simulink library "avionics_T2_lib"  (Simulink 6.6)
undefined symbols (not defined in the file or in its folder): EngineID, Timestep
libraries: aeroutilslib x3, Telemetry_Lib x3, Calibration_Lib x2, simulink x1
settings Model: Creator=amurch  LastModifiedBy=amurch

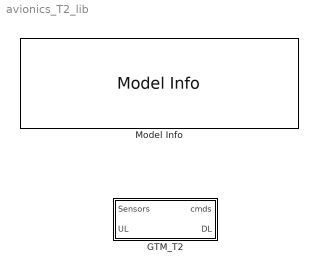
== system avionics_T2_lib ==
  GTM_T2 : Subsystem
  Model Info : simulink/Model-Wide Utilities/Model Info  SystemSampleTime=-1  InitialBlockCM=None  BlockCM=None  Frame=on  DisplayStringWithTags=|  HorizontalTextAlignment=Center  LeftAlignmentValue=0.5  SourceBlockDiagram=avionics_T2_lib  TagMaxNumber=20
      | GTM T2 Avionics Library
      | %<ModelVersion>
      | Las modified by %<LastModifiedBy> on %<LastModificationDate>

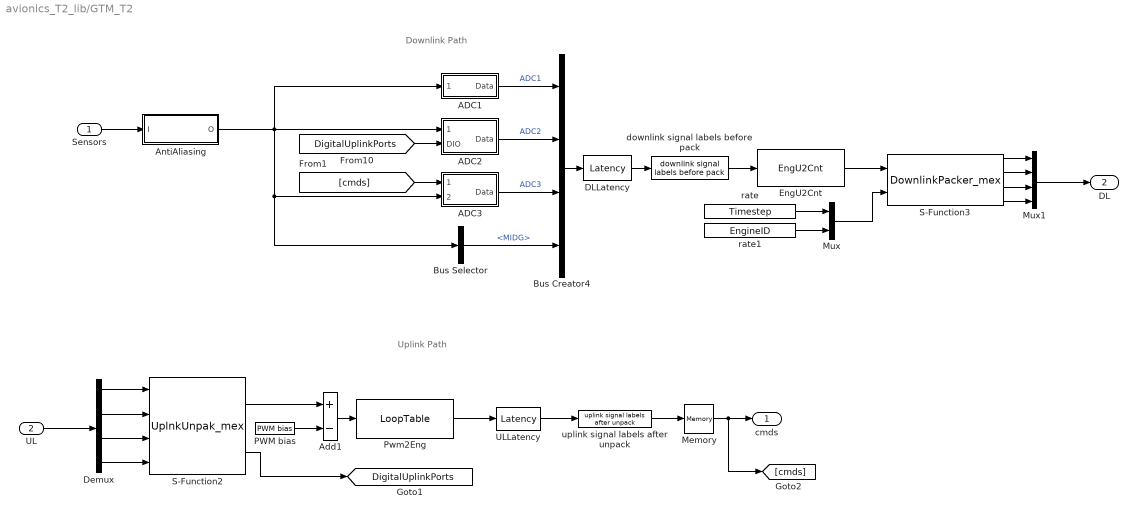
== system avionics_T2_lib/GTM_T2 ==
  note: Downlink Path
  note: Uplink Path
  Sensors : Inport
  UL : Inport  Port=2
  ADC1 : Subsystem
  ADC2 : Subsystem
  ADC3 : Subsystem
  Add1 : Sum  Inputs=+-  OutScaling=2^-10
  AntiAliasing : Subsystem
  Bus Creator4 : BusCreator
  Bus Selector : BusSelector  OutputSignals=MIDG
  DLLatency : aeroutilslib/Latency  SystemSampleTime=-1  Latency=.01  timestep=Timestep
  Demux : Demux
  EngU2Cnt : Calibration_Lib/EngU2Cnt  SystemSampleTime=-1
  Memory : Memory
  Mux : Mux  Inputs=2
  Mux1 : Mux
  PWM bias : Telemetry_Lib/PWM bias  SystemSampleTime=-1
  Pwm2Eng : Calibration_Lib/LoopTable  SystemSampleTime=-1  XTable=UpCals_Pwm  YTable=UpCals_Eng
  S-Function2 : S-Function  FunctionName=UplnkUnpak_mex
  S-Function3 : S-Function  FunctionName=DownlinkPacker_mex
  ULLatency : aeroutilslib/Latency  SystemSampleTime=-1  Latency=.01  timestep=Timestep
  downlink signal labels before pack : Telemetry_Lib/downlink signal labels before pack  SystemSampleTime=-1
  rate : Constant  Value=Timestep
  rate1 : Constant  Value=EngineID
  uplink signal labels after unpack : Telemetry_Lib/uplink signal labels after unpack  SystemSampleTime=-1
  cmds : Outport
  DL : Outport  Port=2
  tag scope: DigitalUplinkPorts=global
  wires:
  S-Function2/1 -> Add1/1
  Add1/1 -> Pwm2Eng/1
  PWM bias/1 -> Add1/2
  [cmds] -> ADC3/1(cmds)
  [DigitalUplinkPorts] -> ADC2/2(DIO)
  DLLatency/1 -> downlink signal labels before pack/1
  downlink signal labels before pack/1 -> EngU2Cnt/1
  ULLatency/1 -> uplink signal labels after unpack/1
  Memory/1 -> [cmds], cmds/1
  Bus Creator4/1 -> DLLatency/1
  Bus Selector/1 -> Bus Creator4/4  "<MIDG>"
  AntiAliasing/1(O) -> Bus Selector/1, ADC3/2(ADC3), ADC2/1(ADC2), ADC1/1(ADC1)
  ADC3/1(Data) -> Bus Creator4/3  "ADC3"
  ADC2/1(Data) -> Bus Creator4/2  "ADC2"
  ADC1/1(Data) -> Bus Creator4/1  "ADC1"
  UL/1 -> Demux/1
  Demux/4 -> S-Function2/4
  Demux/3 -> S-Function2/3
  Demux/2 -> S-Function2/2
  Demux/1 -> S-Function2/1
  uplink signal labels after unpack/1 -> Memory/1
  Pwm2Eng/1 -> ULLatency/1
  S-Function2/2 -> [DigitalUplinkPorts]
  Mux1/1 -> DL/1
  S-Function3/4 -> Mux1/4
  S-Function3/3 -> Mux1/3
  S-Function3/2 -> Mux1/2
  S-Function3/1 -> Mux1/1
  Mux/1 -> S-Function3/2
  rate1/1 -> Mux/2
  rate/1 -> Mux/1
  EngU2Cnt/1 -> S-Function3/1
  Sensors/1 -> AntiAliasing/1(I)

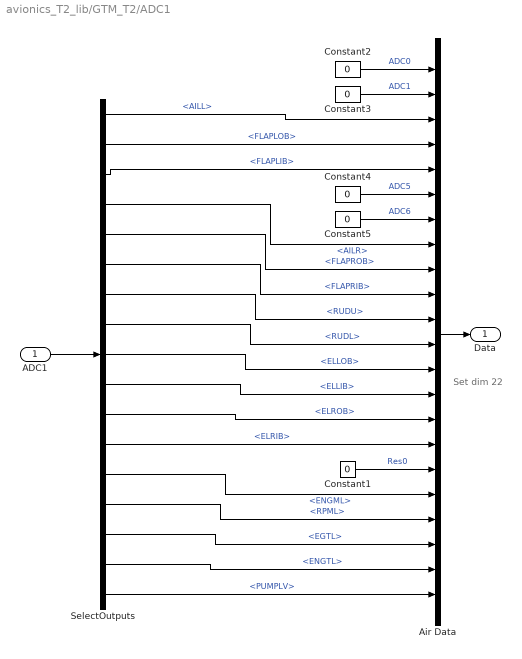
== system avionics_T2_lib/GTM_T2/ADC1 ==
  note: Set dim 22
  ADC1 : Inport
  Air Data : BusCreator  Inputs=22
  Constant{1..5} (5 alike) : Constant  Value=0
  SelectOutputs : BusSelector  OutputSignals=Pots.AILL,Pots.FLAPLOB,Pots.FLAPLIB,Pots.AILR,Pots.FLAPROB,Pots.FLAPRIB,Pots.RUDU,Pots.RUDL,Pots.ELLOB,Pots.ELLIB,Pots.ELROB,Pots.ELRIB,ECUL.ENGML,ECUL.RPML,ECUL.EGTL,ECUL.ENGTL,ECUL.PUMPLV
  Data : Outport  PortDimensions=22
  wires:
  SelectOutputs/17 -> Air Data/22  "<PUMPLV>"
  SelectOutputs/16 -> Air Data/21  "<ENGTL>"
  SelectOutputs/15 -> Air Data/20  "<EGTL>"
  SelectOutputs/14 -> Air Data/19  "<RPML>"
  SelectOutputs/13 -> Air Data/18  "<ENGML>"
  SelectOutputs/12 -> Air Data/16  "<ELRIB>"
  SelectOutputs/11 -> Air Data/15  "<ELROB>"
  SelectOutputs/10 -> Air Data/14  "<ELLIB>"
  SelectOutputs/9 -> Air Data/13  "<ELLOB>"
  SelectOutputs/8 -> Air Data/12  "<RUDL>"
  SelectOutputs/7 -> Air Data/11  "<RUDU>"
  SelectOutputs/6 -> Air Data/10  "<FLAPRIB>"
  SelectOutputs/5 -> Air Data/9  "<FLAPROB>"
  SelectOutputs/4 -> Air Data/8  "<AILR>"
  SelectOutputs/3 -> Air Data/5  "<FLAPLIB>"
  SelectOutputs/2 -> Air Data/4  "<FLAPLOB>"
  SelectOutputs/1 -> Air Data/3  "<AILL>"
  Constant5/1 -> Air Data/7  "ADC6"
  Constant4/1 -> Air Data/6  "ADC5"
  Constant3/1 -> Air Data/2  "ADC1"
  Constant2/1 -> Air Data/1  "ADC0"
  ADC1/1 -> SelectOutputs/1
  Air Data/1 -> Data/1
  Constant1/1 -> Air Data/17  "Res0"

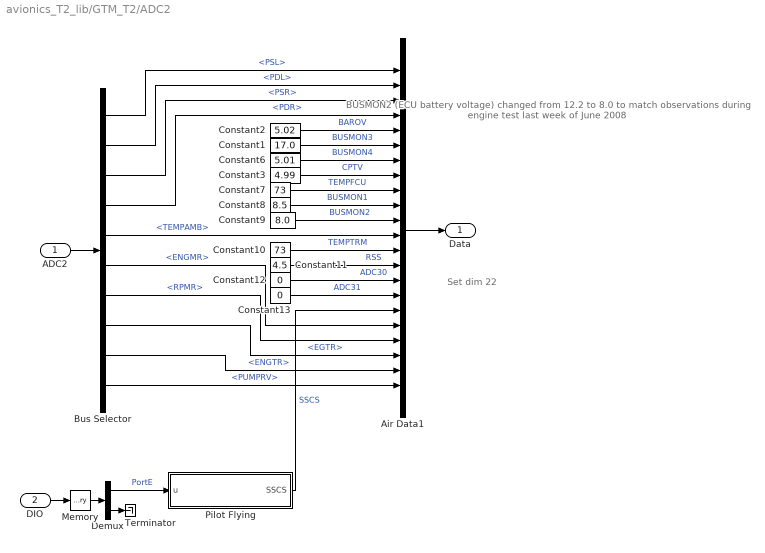
== system avionics_T2_lib/GTM_T2/ADC2 ==
  note: Set dim 22
  note: BUSMON2 (ECU battery voltage)
      | changed from 12.2 to 8.0 to
      | match observations during engine test
      | last week of June 2008
  ADC2 : Inport
  DIO : Inport  Port=2
  Air Data1 : BusCreator  Inputs=22
  Bus Selector : BusSelector  OutputSignals=AirData.PSL,AirData.PDL,AirData.PSR,AirData.PDR,AirData.TEMPAMB,ECUR.ENGMR,ECUR.RPMR,ECUR.EGTR,ECUR.ENGTR,ECUR.PUMPRV
  Constant1 : Constant  Value=17.0
  Constant10 : Constant  Value=73
  Constant11 : Constant  Value=4.5
  Constant12 : Constant  Value=0
  Constant13 : Constant  Value=0
  Constant2 : Constant  Value=5.02
  Constant3 : Constant  Value=4.99
  Constant6 : Constant  Value=5.01
  Constant7 : Constant  Value=73
  Constant8 : Constant  Value=8.5
  Constant9 : Constant  Value=8.0
  Demux : Demux  Outputs=2
  Memory : Memory
  Pilot Flying : Stateflow chart
  Terminator : Terminator
  Data : Outport  PortDimensions=22
  wires:
  Bus Selector/10 -> Air Data1/22  "<PUMPRV>"
  Bus Selector/9 -> Air Data1/21  "<ENGTR>"
  Bus Selector/8 -> Air Data1/20  "<EGTR>"
  Bus Selector/7 -> Air Data1/19  "<RPMR>"
  Bus Selector/6 -> Air Data1/18  "<ENGMR>"
  Memory/1 -> Demux/1
  Demux/1 -> Pilot Flying/1(u)  "PortE"
  Demux/2 -> Terminator/1
  DIO/1 -> Memory/1
  Pilot Flying/1(SSCS) -> Air Data1/17  "SSCS"
  Constant13/1 -> Air Data1/16  "ADC31"
  Constant12/1 -> Air Data1/15  "ADC30"
  Constant11/1 -> Air Data1/14  "RSS"
  Constant10/1 -> Air Data1/13  "TEMPTRM"
  Constant9/1 -> Air Data1/11  "BUSMON2"
  Constant8/1 -> Air Data1/10  "BUSMON1"
  Constant7/1 -> Air Data1/9  "TEMPFCU"
  Constant3/1 -> Air Data1/8  "CPTV"
  Constant6/1 -> Air Data1/7  "BUSMON4"
  Constant1/1 -> Air Data1/6  "BUSMON3"
  Constant2/1 -> Air Data1/5  "BAROV"
  Bus Selector/5 -> Air Data1/12  "<TEMPAMB>"
  Bus Selector/4 -> Air Data1/4  "<PDR>"
  Bus Selector/3 -> Air Data1/3  "<PSR>"
  Bus Selector/2 -> Air Data1/2  "<PDL>"
  Bus Selector/1 -> Air Data1/1  "<PSL>"
  ADC2/1 -> Bus Selector/1
  Air Data1/1 -> Data/1

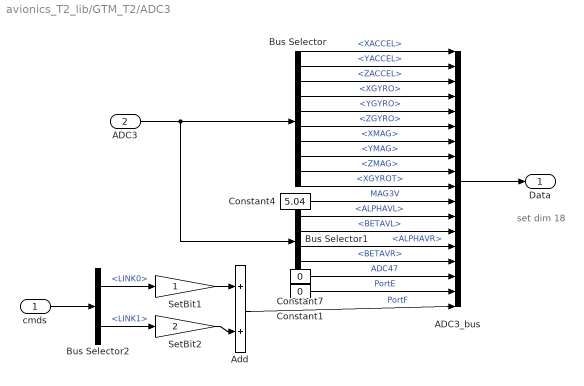
== system avionics_T2_lib/GTM_T2/ADC3 ==
  note: set dim 18
  cmds : Inport
  ADC3 : Inport  Port=2
  ADC3_bus : BusCreator  Inputs=18
  Add : Sum  OutScaling=2^-10
  Bus Selector : BusSelector  OutputSignals=MAG3.XACCEL,MAG3.YACCEL,MAG3.ZACCEL,MAG3.XGYRO,MAG3.YGYRO,MAG3.ZGYRO,MAG3.XMAG,MAG3.YMAG,MAG3.ZMAG,MAG3.XGYROT
  Bus Selector1 : BusSelector  OutputSignals=Vanes.ALPHAVL,Vanes.BETAVL,Vanes.ALPHAVR,Vanes.BETAVR
  Bus Selector2 : BusSelector  OutputSignals=LINK0,LINK1
  Constant1 : Constant  Value=0
  Constant4 : Constant  Value=5.04
  Constant7 : Constant  Value=0
  SetBit1 : Gain
  SetBit2 : Gain  Gain=2
  Data : Outport  PortDimensions=18
  wires:
  SetBit2/1 -> Add/2
  SetBit1/1 -> Add/1
  Bus Selector2/2 -> SetBit2/1  "<LINK1>"
  Bus Selector2/1 -> SetBit1/1  "<LINK0>"
  Bus Selector/9 -> ADC3_bus/9  "<ZMAG>"
  Bus Selector/8 -> ADC3_bus/8  "<YMAG>"
  Bus Selector/7 -> ADC3_bus/7  "<XMAG>"
  Bus Selector/6 -> ADC3_bus/6  "<ZGYRO>"
  Bus Selector/5 -> ADC3_bus/5  "<YGYRO>"
  Bus Selector/4 -> ADC3_bus/4  "<XGYRO>"
  Bus Selector/3 -> ADC3_bus/3  "<ZACCEL>"
  Bus Selector/2 -> ADC3_bus/2  "<YACCEL>"
  Bus Selector/1 -> ADC3_bus/1  "<XACCEL>"
  Bus Selector/10 -> ADC3_bus/10  "<XGYROT>"
  Constant7/1 -> ADC3_bus/16  "ADC47"
  Bus Selector1/4 -> ADC3_bus/15  "<BETAVR>"
  Bus Selector1/3 -> ADC3_bus/14  "<ALPHAVR>"
  Bus Selector1/2 -> ADC3_bus/13  "<BETAVL>"
  Bus Selector1/1 -> ADC3_bus/12  "<ALPHAVL>"
  Constant4/1 -> ADC3_bus/11  "MAG3V"
  ADC3/1 -> Bus Selector1/1, Bus Selector/1
  ADC3_bus/1 -> Data/1
  Constant1/1 -> ADC3_bus/17  "PortE"
  cmds/1 -> Bus Selector2/1
  Add/1 -> ADC3_bus/18  "PortF"

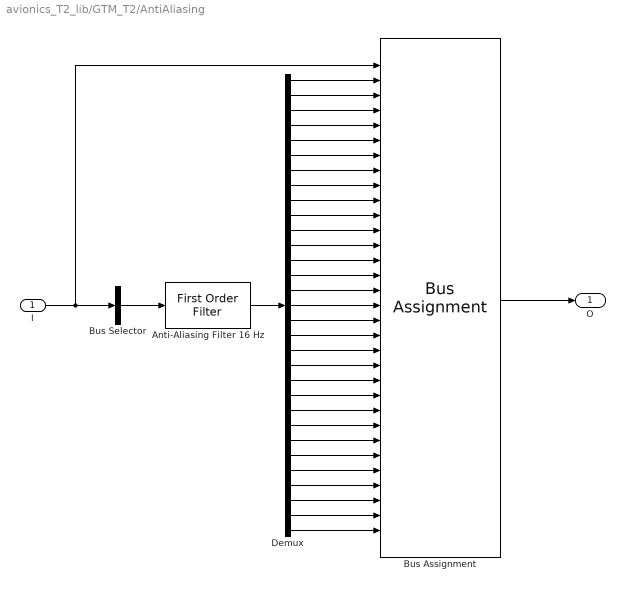
== system avionics_T2_lib/GTM_T2/AntiAliasing ==
  I : Inport
  Anti-Aliasing Filter 16 Hz : aeroutilslib/First Order Filter  SystemSampleTime=-1  tau=1/(32*pi)  timestep=Timestep
  Bus Assignment : BusAssignment  AssignedSignals=Vanes.ALPHAVL,Vanes.BETAVL,Vanes.ALPHAVR,Vanes.BETAVR,AirData.PDL,AirData.PSL,AirData.PDR,AirData.PSR,AirData.TEMPAMB,MAG3.XMAG,MAG3.YMAG,MAG3.ZMAG,MAG3.XGYRO,MAG3.YGYRO,MAG3.ZGYRO,MAG3.XACCEL,MAG3.YACCEL,MAG3.ZACCEL,MAG3.XGYROT,Pots.ELLOB,Pots.ELLIB,Pots.ELROB,Pots.ELRIB,Pots.AILL,Pots.AILR,Pots.RUDU,Pots.RUDL,Pots.FLAPLIB,Pots.FLAPLOB,Pots.FLAPRIB,Pots.FLAPROB
  Bus Selector : BusSelector  OutputSignals=Vanes,AirData,MAG3,Pots  OutputAsBus=on
  Demux : Demux  Outputs=31
  O : Outport
  wires:
  Demux/31 -> Bus Assignment/32
  Demux/30 -> Bus Assignment/31
  Demux/29 -> Bus Assignment/30
  Demux/28 -> Bus Assignment/29
  Demux/27 -> Bus Assignment/28
  Demux/26 -> Bus Assignment/27
  Demux/25 -> Bus Assignment/26
  Demux/24 -> Bus Assignment/25
  Demux/23 -> Bus Assignment/24
  Demux/22 -> Bus Assignment/23
  Demux/21 -> Bus Assignment/22
  Demux/20 -> Bus Assignment/21
  Demux/19 -> Bus Assignment/20
  Demux/18 -> Bus Assignment/19
  Demux/17 -> Bus Assignment/18
  Demux/16 -> Bus Assignment/17
  Demux/15 -> Bus Assignment/16
  Demux/14 -> Bus Assignment/15
  Demux/13 -> Bus Assignment/14
  Demux/12 -> Bus Assignment/13
  Demux/11 -> Bus Assignment/12
  Demux/10 -> Bus Assignment/11
  Demux/9 -> Bus Assignment/10
  Demux/8 -> Bus Assignment/9
  Demux/7 -> Bus Assignment/8
  Demux/6 -> Bus Assignment/7
  Demux/5 -> Bus Assignment/6
  Demux/4 -> Bus Assignment/5
  Demux/3 -> Bus Assignment/4
  Demux/2 -> Bus Assignment/3
  Demux/1 -> Bus Assignment/2
  Bus Assignment/1 -> O/1
  Anti-Aliasing Filter 16 Hz/1 -> Demux/1
  Bus Selector/1 -> Anti-Aliasing Filter 16 Hz/1
  I/1 -> Bus Assignment/1, Bus Selector/1

== matlab function GTM_T2/ADC2/Pilot Flying ==
  data: u input inherited; SSCS output inherited
function SSCS = setSSCS(u)
% This block supports an embeddable subset of the MATLAB language.
% See the help menu for details. 

SSCS = double(0);
RPf = uint8(0);
RPf = bitget(u,8);
if RPf==1
    SSCS = 6.0;  %research pilot flying (SSCS)
else
    SSCS = 4.0;  %safety pilot flying  (SSCS)
end
